simulink model "sim1"  (R2023a)
settings: Solver=VariableStepAuto  StartTime=0.0  StopTime=20  FixedStep=0.000001  RelTol=1e-3
values from neighbouring files (symbols this model uses):
  dt1 = 1/fs1    (= 0.2)    [sim_data2.m]
  dt2 = 1/fs2    (= 0.0333333333333)    [sim_data2.m]
  dt3 = 1/fs3    (= 0.01)    [sim_data2.m]
undefined symbols (not defined in the file or in its folder): Ac, Ad1, Ad2, Ad3, Bc, Bd1, Bd2, Bd3, Cc, Cd1, Cd2, Cd3, Dc, Dd1, Dd2, Dd3, S, W
settings Model: Creator=ozar  LastModifiedBy=ozar

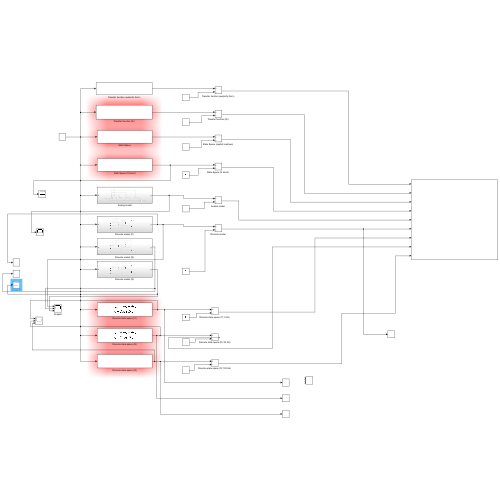
[thumbnail: Simulink's stored preview of the top-level diagram]
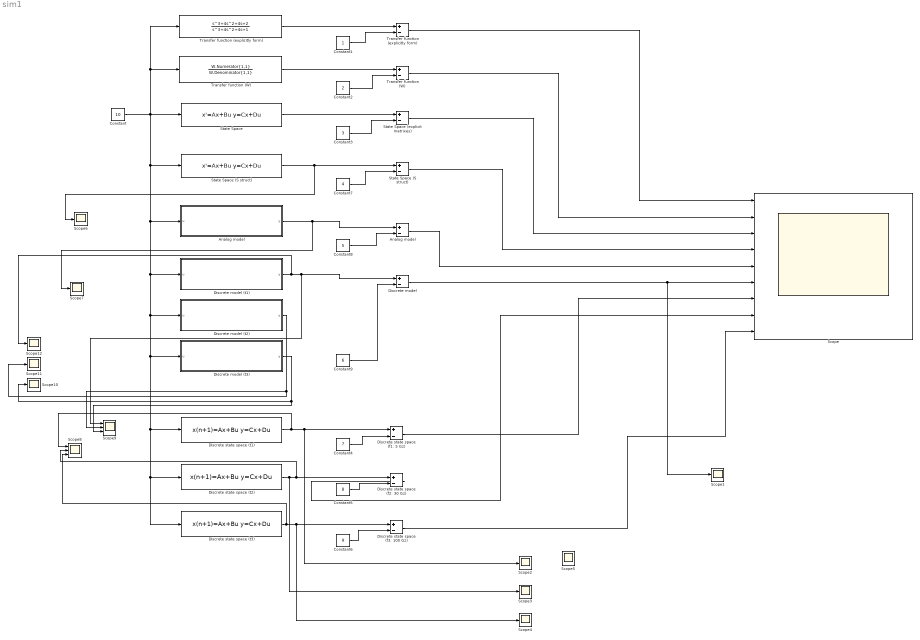
== system sim1 ==
  Analog model : Subsystem
  "Analog model " : Sum  Inputs=+-
  Constant : Constant  Value=10
  Constant1 : Constant
  Constant2 : Constant  Value=2
  Constant3 : Constant  Value=3
  Constant4 : Constant  Value=7
  Constant5 : Constant  Value=8
  Constant6 : Constant  Value=9
  Constant7 : Constant  Value=4
  Constant8 : Constant  Value=5
  Constant9 : Constant  Value=6
  "Discrete model " : Sum  Inputs=+-
  Discrete model (t1) : Subsystem
  Discrete model (t2) : Subsystem
  Discrete model (t3) : Subsystem
  "Discrete state space (f1: 5 Gz) " : Sum  Inputs=+-
  "Discrete state space (f2: 30 Gz) " : Sum  Inputs=+-
  "Discrete state space (f3: 100 Gz) " : Sum  Inputs=+-
  Discrete state space (t1) : DiscreteStateSpace  A=Ad1  B=Bd1  C=Cd1  D=Dd1  SampleTime=dt1
  Discrete state space (t2) : DiscreteStateSpace  A=Ad2  B=Bd2  C=Cd2  D=Dd2  SampleTime=dt2
  Discrete state space (t3) : DiscreteStateSpace  A=Ad3  B=Bd3  C=Cd3  D=Dd3  SampleTime=dt3
  Scope : Scope  NumInputPorts=9
  Scope{1..4,6..7,10..12} (9 alike) : Scope
  Scope5 : Scope  NumInputPorts=3
  Scope8 : Scope  NumInputPorts=3
  Scope9 : Scope  NumInputPorts=3
  State Space : StateSpace  A=Ac  B=Bc  C=Cc  D=Dc  InitialCondition=0
  State Space (S struct) : StateSpace  A=S.A  B=S.B  C=S.C  D=S.D  InitialCondition=0
  "State Space (S struct) " : Sum  Inputs=+-
  "State Space (explicit matrixes) " : Sum  Inputs=+-
  Transfer function (W) : TransferFcn  Numerator=W.Numerator{1,1}  Denominator=W.Denominator{1,1}
  "Transfer function (W) " : Sum  Inputs=+-
  Transfer function (explicitly form) : TransferFcn  Numerator=[1 4 4 2]  Denominator=[1 4 4 1]
  "Transfer function (explicitly form) " : Sum  Inputs=+-
  wires:
  Transfer function (explicitly form)/1 -> "Transfer function (explicitly form) "/1
  Constant1/1 -> "Transfer function (explicitly form) "/2
  "Transfer function (explicitly form) "/1 -> Scope/1
  Constant2/1 -> "Transfer function (W) "/2
  Transfer function (W)/1 -> "Transfer function (W) "/1
  "Transfer function (W) "/1 -> Scope/2
  Constant3/1 -> "State Space (explicit matrixes) "/2
  State Space/1 -> "State Space (explicit matrixes) "/1
  "State Space (explicit matrixes) "/1 -> Scope/3
  Constant4/1 -> "Discrete state space (f1: 5 Gz) "/2
  Discrete state space (t1)/1 -> Scope8/1, Scope2/1, "Discrete state space (f1: 5 Gz) "/1
  "Discrete state space (f1: 5 Gz) "/1 -> Scope/7
  Constant5/1 -> "Discrete state space (f2: 30 Gz) "/2
  Discrete state space (t2)/1 -> Scope3/1, Scope8/2, "Discrete state space (f2: 30 Gz) "/1
  "Discrete state space (f2: 30 Gz) "/1 -> Scope/8
  "Discrete state space (f3: 100 Gz) "/1 -> Scope/9
  Constant6/1 -> "Discrete state space (f3: 100 Gz) "/2
  Discrete state space (t3)/1 -> Scope8/3, Scope4/1, "Discrete state space (f3: 100 Gz) "/1
  State Space (S struct)/1 -> Scope6/1, "State Space (S struct) "/1
  Constant7/1 -> "State Space (S struct) "/2
  "State Space (S struct) "/1 -> Scope/4
  Constant8/1 -> "Analog model "/2
  Discrete model (t1)/1(y) -> Scope12/1, Scope9/1, "Discrete model "/1
  Constant9/1 -> "Discrete model "/2
  Analog model/1(y) -> Scope7/1, "Analog model "/1
  "Analog model "/1 -> Scope/5
  "Discrete model "/1 -> Scope1/1, Scope/6
  Constant/1 -> Transfer function (explicitly form)/1, Transfer function (W)/1, State Space (S struct)/1, Discrete model (t3)/1(u), Discrete state space (t3)/1, Discrete state space (t2)/1, Discrete state space (t1)/1, Discrete model (t2)/1(u), Discrete model (t1)/1(u), Analog model/1(u), State Space/1
  Discrete model (t3)/1(y) -> Scope10/1, Scope9/3
  Discrete model (t2)/1(y) -> Scope11/1, Scope9/2

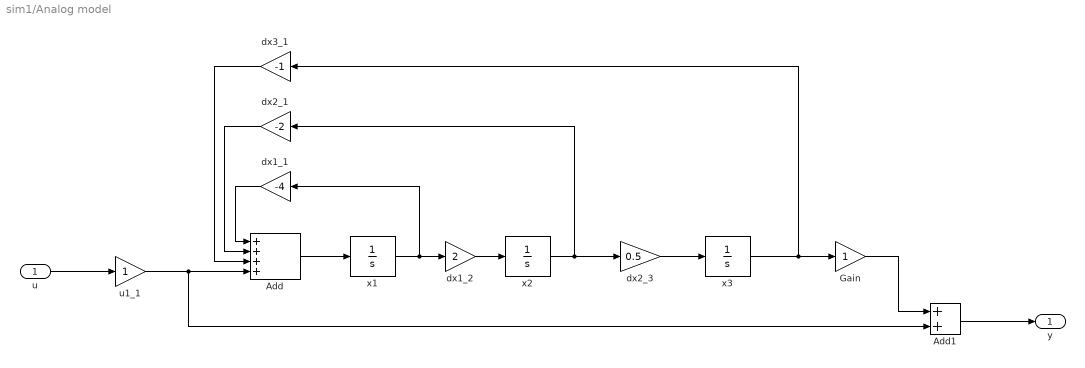
== system sim1/Analog model ==
  u : Inport
  Add : Sum  Inputs=++++
  Add1 : Sum
  Gain : Gain
  dx1_1 : Gain  Gain=-4
  dx1_2 : Gain  Gain=2
  dx2_1 : Gain  Gain=-2
  dx2_3 : Gain  Gain=0.5
  dx3_1 : Gain  Gain=-1
  u1_1 : Gain
  x1 : Integrator
  x2 : Integrator
  x3 : Integrator
  y : Outport
  wires:
  dx1_1/1 -> Add/1
  dx2_1/1 -> Add/2
  dx3_1/1 -> Add/3
  Add/1 -> x1/1
  u/1 -> u1_1/1
  x1/1 -> dx1_1/1, dx1_2/1
  u1_1/1 -> Add1/2, Add/4
  x2/1 -> dx2_3/1, dx2_1/1
  x3/1 -> Gain/1, dx3_1/1
  dx1_2/1 -> x2/1
  dx2_3/1 -> x3/1
  Gain/1 -> Add1/1
  Add1/1 -> y/1

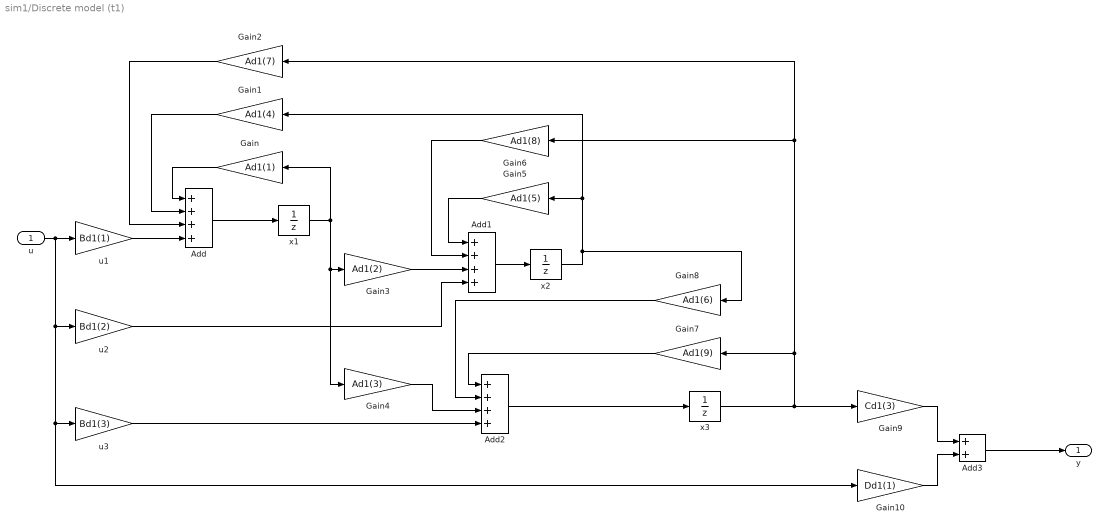
== system sim1/Discrete model (t1) ==
  u : Inport
  Add : Sum  Inputs=++++
  Add1 : Sum  Inputs=++++
  Add2 : Sum  Inputs=++++
  Add3 : Sum
  Gain : Gain  Gain=Ad1(1)
  Gain1 : Gain  Gain=Ad1(4)
  Gain10 : Gain  Gain=Dd1(1)
  Gain2 : Gain  Gain=Ad1(7)
  Gain3 : Gain  Gain=Ad1(2)
  Gain4 : Gain  Gain=Ad1(3)
  Gain5 : Gain  Gain=Ad1(5)
  Gain6 : Gain  Gain=Ad1(8)
  Gain7 : Gain  Gain=Ad1(9)
  Gain8 : Gain  Gain=Ad1(6)
  Gain9 : Gain  Gain=Cd1(3)
  u1 : Gain  Gain=Bd1(1)
  u2 : Gain  Gain=Bd1(2)
  u3 : Gain  Gain=Bd1(3)
  x1 : UnitDelay  SampleTime=dt1  HasFrameUpgradeWarning=on
  x2 : UnitDelay  SampleTime=dt1  HasFrameUpgradeWarning=on
  x3 : UnitDelay  SampleTime=dt1  HasFrameUpgradeWarning=on
  y : Outport
  wires:
  u/1 -> Gain10/1, u3/1, u2/1, u1/1
  u1/1 -> Add/4
  Add/1 -> x1/1
  x1/1 -> Gain4/1, Gain3/1, Gain/1
  Gain/1 -> Add/1
  Gain1/1 -> Add/2
  Gain2/1 -> Add/3
  x2/1 -> Gain1/1, Gain5/1, Gain8/1
  x3/1 -> Gain9/1, Gain7/1, Gain6/1, Gain2/1
  Add1/1 -> x2/1
  u2/1 -> Add1/4
  Gain3/1 -> Add1/3
  Gain5/1 -> Add1/1
  Gain6/1 -> Add1/2
  u3/1 -> Add2/4
  Gain4/1 -> Add2/3
  Gain7/1 -> Add2/1
  Add2/1 -> x3/1
  Gain8/1 -> Add2/2
  Gain9/1 -> Add3/1
  Gain10/1 -> Add3/2
  Add3/1 -> y/1

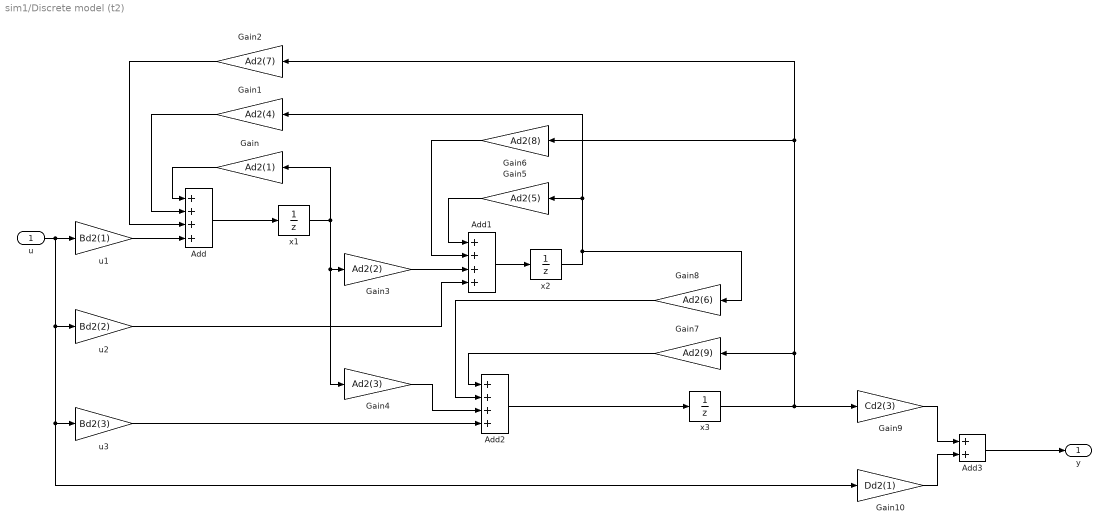
== system sim1/Discrete model (t2) ==
  u : Inport
  Add : Sum  Inputs=++++
  Add1 : Sum  Inputs=++++
  Add2 : Sum  Inputs=++++
  Add3 : Sum
  Gain : Gain  Gain=Ad2(1)
  Gain1 : Gain  Gain=Ad2(4)
  Gain10 : Gain  Gain=Dd2(1)
  Gain2 : Gain  Gain=Ad2(7)
  Gain3 : Gain  Gain=Ad2(2)
  Gain4 : Gain  Gain=Ad2(3)
  Gain5 : Gain  Gain=Ad2(5)
  Gain6 : Gain  Gain=Ad2(8)
  Gain7 : Gain  Gain=Ad2(9)
  Gain8 : Gain  Gain=Ad2(6)
  Gain9 : Gain  Gain=Cd2(3)
  u1 : Gain  Gain=Bd2(1)
  u2 : Gain  Gain=Bd2(2)
  u3 : Gain  Gain=Bd2(3)
  x1 : UnitDelay  SampleTime=dt2  HasFrameUpgradeWarning=on
  x2 : UnitDelay  SampleTime=dt2  HasFrameUpgradeWarning=on
  x3 : UnitDelay  SampleTime=dt2  HasFrameUpgradeWarning=on
  y : Outport
  wires:
  Add3/1 -> y/1
  Gain10/1 -> Add3/2
  Gain9/1 -> Add3/1
  Gain8/1 -> Add2/2
  Add2/1 -> x3/1
  Gain7/1 -> Add2/1
  Gain4/1 -> Add2/3
  u3/1 -> Add2/4
  Gain6/1 -> Add1/2
  Gain5/1 -> Add1/1
  Gain3/1 -> Add1/3
  u2/1 -> Add1/4
  Add1/1 -> x2/1
  x3/1 -> Gain2/1, Gain6/1, Gain7/1, Gain9/1
  x2/1 -> Gain8/1, Gain5/1, Gain1/1
  Gain2/1 -> Add/3
  Gain1/1 -> Add/2
  Gain/1 -> Add/1
  x1/1 -> Gain/1, Gain3/1, Gain4/1
  Add/1 -> x1/1
  u1/1 -> Add/4
  u/1 -> u1/1, u2/1, u3/1, Gain10/1

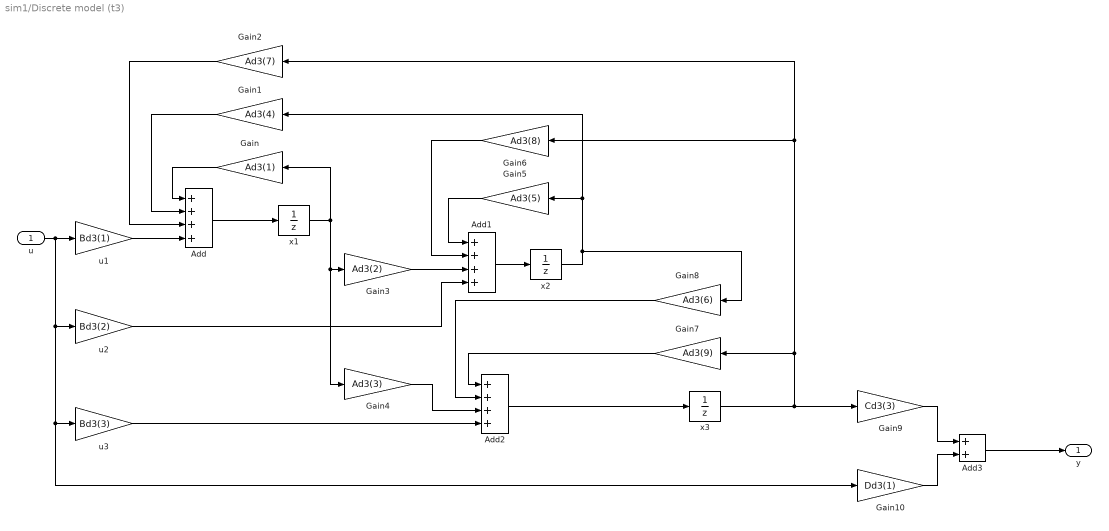
== system sim1/Discrete model (t3) ==
  u : Inport
  Add : Sum  Inputs=++++
  Add1 : Sum  Inputs=++++
  Add2 : Sum  Inputs=++++
  Add3 : Sum
  Gain : Gain  Gain=Ad3(1)
  Gain1 : Gain  Gain=Ad3(4)
  Gain10 : Gain  Gain=Dd3(1)
  Gain2 : Gain  Gain=Ad3(7)
  Gain3 : Gain  Gain=Ad3(2)
  Gain4 : Gain  Gain=Ad3(3)
  Gain5 : Gain  Gain=Ad3(5)
  Gain6 : Gain  Gain=Ad3(8)
  Gain7 : Gain  Gain=Ad3(9)
  Gain8 : Gain  Gain=Ad3(6)
  Gain9 : Gain  Gain=Cd3(3)
  u1 : Gain  Gain=Bd3(1)
  u2 : Gain  Gain=Bd3(2)
  u3 : Gain  Gain=Bd3(3)
  x1 : UnitDelay  SampleTime=dt3  HasFrameUpgradeWarning=on
  x2 : UnitDelay  SampleTime=dt3  HasFrameUpgradeWarning=on
  x3 : UnitDelay  SampleTime=dt3  HasFrameUpgradeWarning=on
  y : Outport
  wires:
  u/1 -> Gain10/1, u3/1, u2/1, u1/1
  u1/1 -> Add/4
  Add/1 -> x1/1
  x1/1 -> Gain4/1, Gain3/1, Gain/1
  Gain/1 -> Add/1
  Gain1/1 -> Add/2
  Gain2/1 -> Add/3
  x2/1 -> Gain1/1, Gain5/1, Gain8/1
  x3/1 -> Gain9/1, Gain7/1, Gain6/1, Gain2/1
  Add1/1 -> x2/1
  u2/1 -> Add1/4
  Gain3/1 -> Add1/3
  Gain5/1 -> Add1/1
  Gain6/1 -> Add1/2
  u3/1 -> Add2/4
  Gain4/1 -> Add2/3
  Gain7/1 -> Add2/1
  Add2/1 -> x3/1
  Gain8/1 -> Add2/2
  Gain9/1 -> Add3/1
  Gain10/1 -> Add3/2
  Add3/1 -> y/1
